simulink model "lab7_1"  (R2013b)
settings: Solver=ode45  StartTime=0.0  StopTime=200  RelTol=1e-3
libraries: commanapbnd3 x4
settings Model: Creator=Kseniya  LastModifiedBy=Kseniya

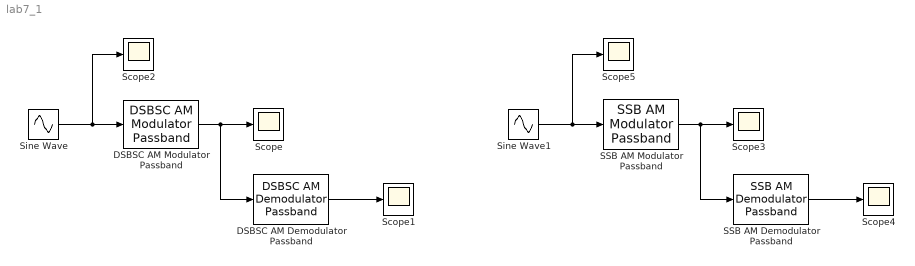
== system lab7_1 ==
  DSBSC AM Demodulator Passband : commanapbnd3/DSBSC AM Demodulator Passband  Fc=5  Ph=0  method=Butterworth  n=4  cf=0.1  Rp=0.1  Rs=50
  DSBSC AM Modulator Passband : commanapbnd3/DSBSC AM Modulator Passband  Fc=5  Ph=0
  SSB AM Demodulator Passband : commanapbnd3/SSB AM Demodulator Passband  Fc=5  Ph=0  method=Butterworth  n=4  cf=1  Rp=0.1  Rs=50
  SSB AM Modulator Passband : commanapbnd3/SSB AM Modulator Passband  Fc=5  Ph=0  Sd=Upper  Ho=50
  Scope{,1..5} (6 alike) : Scope
      Scope2 settings: SaveName=ScopeData2
      Scope3 settings: SaveName=ScopeData3
      Scope4 settings: SaveName=ScopeData4
      Scope5 settings: SaveName=ScopeData5
  Sine Wave : Sin  SampleTime=1/200
  Sine Wave1 : Sin  SampleTime=1/200
  wires:
  Sine Wave/1 -> DSBSC AM Modulator Passband/1, Scope2/1
  DSBSC AM Modulator Passband/1 -> DSBSC AM Demodulator Passband/1, Scope/1
  DSBSC AM Demodulator Passband/1 -> Scope1/1
  Sine Wave1/1 -> SSB AM Modulator Passband/1, Scope5/1
  SSB AM Modulator Passband/1 -> SSB AM Demodulator Passband/1, Scope3/1
  SSB AM Demodulator Passband/1 -> Scope4/1
